simulink model "prob4"  (R2020b)
settings: Solver=VariableStepAuto  StartTime=0.0  StopTime=10.0  RelTol=1e-3
settings Model: Creator=Admin  LastModifiedBy=Admin

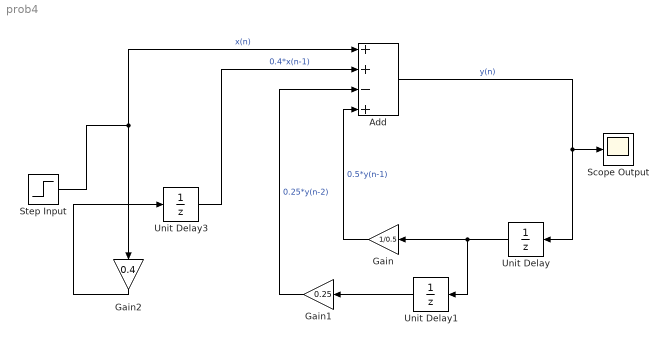
== system prob4 ==
  Add : Sum  Inputs=++-+
  Gain : Gain  Gain=1/0.5
  Gain1 : Gain  Gain=0.25
  Gain2 : Gain  Gain=0.4
  Scope Output : Scope
  Step Input : Step  SampleTime=0
  Unit Delay : UnitDelay  SampleTime=-1  HasFrameUpgradeWarning=on
  Unit Delay1 : UnitDelay  SampleTime=-1  HasFrameUpgradeWarning=on
  Unit Delay3 : UnitDelay  SampleTime=-1  HasFrameUpgradeWarning=on
  wires:
  Gain/1 -> Add/4  "0.5*y(n-1)"
  Add/1 -> Unit Delay/1, Scope Output/1  "y(n)"
  Unit Delay1/1 -> Gain1/1
  Unit Delay/1 -> Unit Delay1/1, Gain/1
  Step Input/1 -> Add/1, Gain2/1  "x(n)"
  Gain1/1 -> Add/3  "0.25*y(n-2)"
  Unit Delay3/1 -> Add/2  "0.4*x(n-1)"
  Gain2/1 -> Unit Delay3/1
